simulink model "regler_trottel_framkoppling_img"  (R2012b)
settings: Solver=ode45  StartTime=0.0  StopTime=10.0  RelTol=1e-3
values from neighbouring files (symbols this model uses):
  a_1 = X(1)    [Init_Project1.m]
  a_2 = X(2)    [Init_Project1.m]
  a_3 = X(3)    [Init_Project1.m]
  gamma_air = 1.3    [Init_Project1.m]
  n_cyl = 4    [Init_Project1.m]
  n_r = 2    [Init_Project1.m]    (also in Init_Project2.m)
  n_vol_parameters = C\D    [Init_Project1.m]
  R_air = 280    [Init_Project1.m]
  T_ic = 1    [Init_Project2.m]
  T_im = mean(T_im)    [Init_Project1.m]
  V_d = 2*a*pi*B^2/4    (= 0.000572555261117)    [Init_Project1.m]    (also in Init_Project2.m = B^2/4*pi*s)
undefined symbols (not defined in the file or in its folder): epsilon, Newton, Raphson
settings Model: Creator=rasme879  LastModifiedBy=rasme879

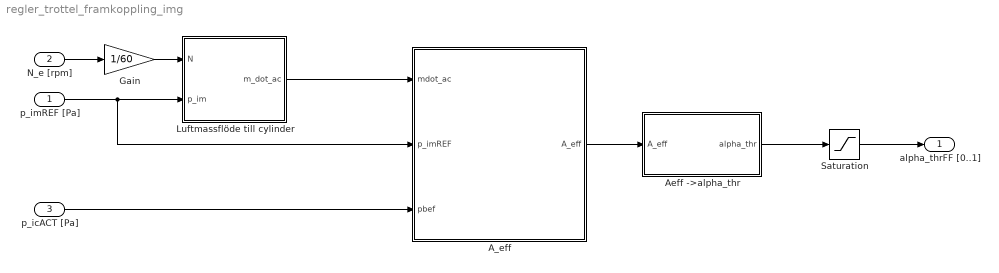
== system regler_trottel_framkoppling_img ==
  p_imREF [Pa] : Inport
  N_e [rpm] : Inport  Port=2
  p_icACT [Pa] : Inport  Port=3
  "A_eff " : Subsystem
  Aeff ->alpha_thr : Subsystem
  Gain : Gain  Gain=1/60
  Luftmassflöde till cylinder : Subsystem
  Saturation : Saturate  UpperLimit=1  LowerLimit=0
  alpha_thrFF [0..1] : Outport
  wires:
  p_imREF [Pa]/1 -> "A_eff "/2(p_imREF), Luftmassflöde till cylinder/2(p_im)
  Luftmassflöde till cylinder/1(m_dot_ac) -> "A_eff "/1(mdot_ac)
  p_icACT [Pa]/1 -> "A_eff "/3(pbef)
  "A_eff "/1(A_eff) -> Aeff ->alpha_thr/1(A_eff)
  Aeff ->alpha_thr/1(alpha_thr) -> Saturation/1
  N_e [rpm]/1 -> Gain/1
  Gain/1 -> Luftmassflöde till cylinder/1(N)
  Saturation/1 -> alpha_thrFF [0..1]/1

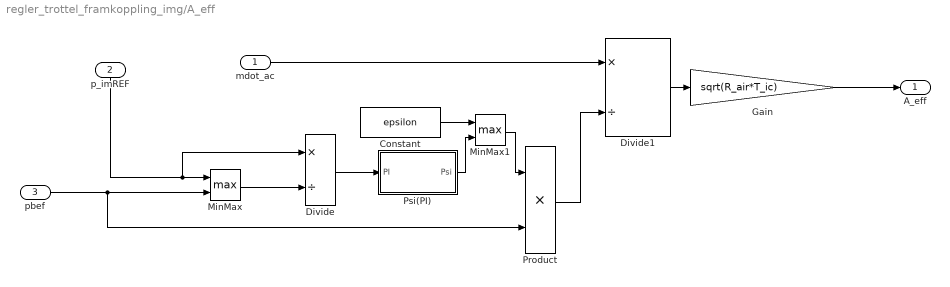
== system regler_trottel_framkoppling_img/A_eff  ==
  mdot_ac : Inport
  p_imREF : Inport  Port=2
  pbef : Inport  Port=3
  Constant : Constant  Value=epsilon
  Divide : Product  Inputs=*/
  Divide1 : Product  Inputs=*/
  Gain : Gain  Gain=sqrt(R_air*T_ic)
  MinMax : MinMax  Function=max  Inputs=2
  MinMax1 : MinMax  Function=max  Inputs=2
  Product : Product  RndMeth=Zero
  Psi(PI) : Subsystem
  A_eff : Outport
  wires:
  Divide/1 -> Psi(PI)/1(PI)
  MinMax/1 -> Divide/2
  Divide1/1 -> Gain/1
  Product/1 -> Divide1/2
  p_imREF/1 -> Divide/1, MinMax/1
  Gain/1 -> A_eff/1
  pbef/1 -> Product/2, MinMax/2
  Psi(PI)/1(Psi) -> MinMax1/2
  mdot_ac/1 -> Divide1/1
  Constant/1 -> MinMax1/1
  MinMax1/1 -> Product/1

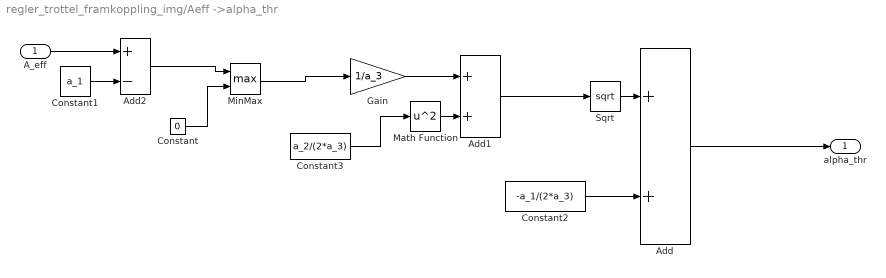
== system regler_trottel_framkoppling_img/Aeff ->alpha_thr ==
  A_eff : Inport
  Add : Sum
  Add1 : Sum
  Add2 : Sum  Inputs=+-
  Constant : Constant  Value=0
  Constant1 : Constant  Value=a_1
  Constant2 : Constant  Value=-a_1/(2*a_3)
  Constant3 : Constant  Value=a_2/(2*a_3)
  Gain : Gain  Gain=1/a_3
  Math Function : Math  Operator=square  SaturateOnIntegerOverflow=on
  MinMax : MinMax  Function=max  Inputs=2
  Sqrt : Sqrt  SaturateOnIntegerOverflow=on
  alpha_thr : Outport
  wires:
  Constant1/1 -> Add2/2
  Gain/1 -> Add1/1
  Sqrt/1 -> Add/1
  Constant2/1 -> Add/2
  Math Function/1 -> Add1/2
  A_eff/1 -> Add2/1
  Constant3/1 -> Math Function/1
  Add/1 -> alpha_thr/1
  Add1/1 -> Sqrt/1
  Constant/1 -> MinMax/2
  Add2/1 -> MinMax/1
  MinMax/1 -> Gain/1

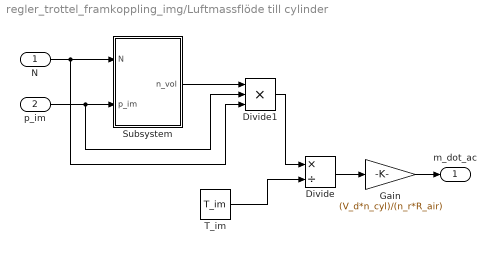
== system regler_trottel_framkoppling_img/Luftmassflöde till cylinder ==
  N : Inport
  p_im : Inport  Port=2
  Divide : Product  Inputs=*/
  Divide1 : Product  Inputs=***
  Gain : Gain  Gain=(V_d*n_cyl)/(n_r*R_air)
  Subsystem : Subsystem
  T_im : Constant  Value=T_im
  m_dot_ac : Outport
  wires:
  N/1 -> Divide1/3, Subsystem/1(N)
  p_im/1 -> Divide1/2, Subsystem/2(p_im)
  Subsystem/1(n_vol) -> Divide1/1
  Divide1/1 -> Divide/1
  Divide/1 -> Gain/1
  Gain/1 -> m_dot_ac/1
  T_im/1 -> Divide/2

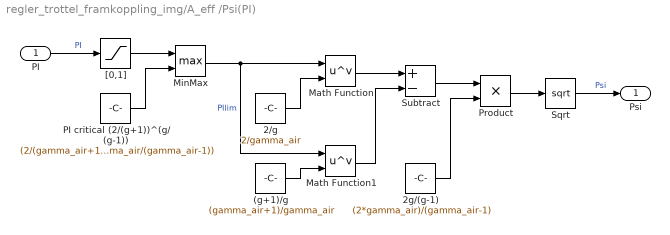
== system regler_trottel_framkoppling_img/A_eff /Psi(PI) ==
  PI : Inport
  (g+1)/g : Constant  Value=(gamma_air+1)/gamma_air
  2/g : Constant  Value=2/gamma_air
  2g/(g-1) : Constant  Value=(2*gamma_air)/(gamma_air-1)
  Math Function : Math  Operator=pow  SaturateOnIntegerOverflow=on
  Math Function1 : Math  Operator=pow  SaturateOnIntegerOverflow=on
  MinMax : MinMax  Function=max  Inputs=2
  PI critical (2/(g+1))^(g/(g-1)) : Constant  Value=(2/(gamma_air+1))^(gamma_air/(gamma_air-1))
  Product : Product  RndMeth=Zero
  Sqrt : Sqrt  AlgorithmType=Newton-Raphson  SaturateOnIntegerOverflow=on
  Subtract : Sum  Inputs=+-
  "[0,1]" : Saturate  UpperLimit=1  LowerLimit=0
  Psi : Outport
  wires:
  PI/1 -> "[0,1]"/1  "PI"
  PI critical (2/(g+1))^(g/(g-1))/1 -> MinMax/2
  MinMax/1 -> Math Function/1, Math Function1/1  "PIlim"
  2/g/1 -> Math Function/2
  (g+1)/g/1 -> Math Function1/2
  "[0,1]"/1 -> MinMax/1
  Math Function/1 -> Subtract/1
  Math Function1/1 -> Subtract/2
  Subtract/1 -> Product/1
  2g/(g-1)/1 -> Product/2
  Product/1 -> Sqrt/1
  Sqrt/1 -> Psi/1  "Psi"

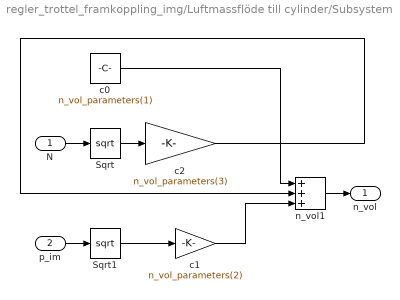
== system regler_trottel_framkoppling_img/Luftmassflöde till cylinder/Subsystem ==
  N : Inport
  p_im : Inport  Port=2
  Sqrt : Sqrt  SaturateOnIntegerOverflow=on
  Sqrt1 : Sqrt  SaturateOnIntegerOverflow=on
  c0 : Constant  Value=n_vol_parameters(1)
  c1 : Gain  Gain=n_vol_parameters(2)
  c2 : Gain  Gain=n_vol_parameters(3)
  n_vol1 : Sum  Inputs=+++
  n_vol : Outport
  wires:
  Sqrt/1 -> c2/1
  Sqrt1/1 -> c1/1
  c0/1 -> n_vol1/1
  c2/1 -> n_vol1/2
  c1/1 -> n_vol1/3
  N/1 -> Sqrt/1
  n_vol1/1 -> n_vol/1
  p_im/1 -> Sqrt1/1
